simulink model "ecse563_part1c_model"  (R2025a)
settings: Solver=VariableStepAuto  StartTime=0.0  StopTime=30  RelTol=1e-3
settings Model: Creator=aliseifeldin  LastModifiedBy=aliseifeldin

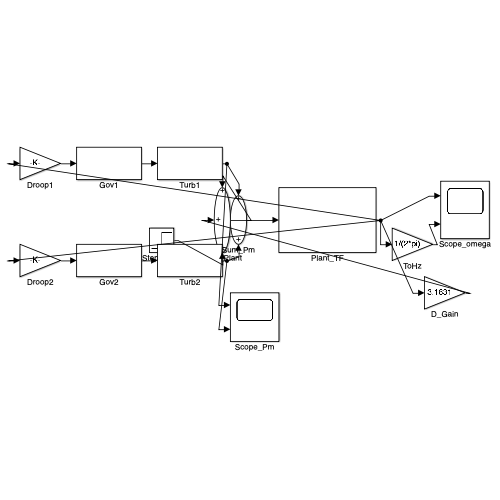
[thumbnail: Simulink's stored preview of the top-level diagram]
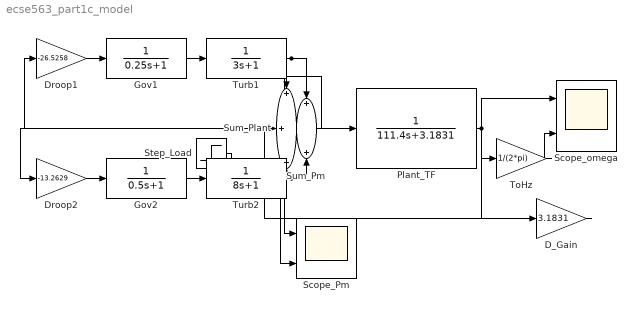
== system ecse563_part1c_model ==
  D_Gain : Gain  Gain=3.1831
  Droop1 : Gain  Gain=-26.5258
  Droop2 : Gain  Gain=-13.2629
  Gov1 : TransferFcn  Numerator=1  Denominator=[0.25 1]
  Gov2 : TransferFcn  Numerator=1  Denominator=[0.5 1]
  Plant_TF : TransferFcn  Numerator=1  Denominator=[111.4 3.1831]
  Scope_Pm : Scope  NumInputPorts=2
  Scope_omega : Scope  NumInputPorts=2
  Step_Load : Step  Time=0  After=100  SampleTime=0
  Sum_Plant : Sum  Inputs=++-
  Sum_Pm : Sum
  ToHz : Gain  Gain=1/(2*pi)
  Turb1 : TransferFcn  Numerator=1  Denominator=[3 1]
  Turb2 : TransferFcn  Numerator=1  Denominator=[8 1]
  wires:
  Plant_TF/1 -> ToHz/1, Droop1/1, Droop2/1, Scope_omega/1, D_Gain/1
  ToHz/1 -> Scope_omega/2
  Droop1/1 -> Gov1/1
  Gov1/1 -> Turb1/1
  Turb1/1 -> Sum_Pm/1, Scope_Pm/1
  Droop2/1 -> Gov2/1
  Gov2/1 -> Turb2/1
  Turb2/1 -> Sum_Pm/2, Scope_Pm/2
  Sum_Pm/1 -> Sum_Plant/1
  D_Gain/1 -> Sum_Plant/2
  Step_Load/1 -> Sum_Plant/3
  Sum_Plant/1 -> Plant_TF/1
